simulink model "quadrotor_linear_ADRC"  (R2018b)
settings: Solver=VariableStepAuto  StartTime=0.0  StopTime=300  RelTol=1e-3
InitFcn:
  | %%%%%%%%%%%%%%%%%%%%%%%%%
  | %                     TUNABLE PARAMETERS                 %
  | %    (ORDER, SETTLING TIME, ESO GAIN AND B0)  %
  | %%%%%%%%%%%%%%%%%%%%%%%%%
  | order = 2;                     % ADRC order
  | ts = 5;                        % Desired settling time
  | b0 = 1;                         % b0 parameter
  | eso_gain = 8;                % ESO Dynamic related to closed-loop poles
  | 
  | %%%%%%%%%%%%%%%%%%%%%%%%%
  | %                                 ADRC                               %
  | %      (CONTROLLER GAINS AND ESO MATRIXES)    %
  | %%%%%%%%%%%%%%%%%%%%%%%%%
  | s_cl = 4/ts;                           % Closed-loop system poles
  | s_eso = eso_gain * s_cl;        % ESO poles
  | pole = [1 s_cl];                     % Base polynomial to calculate
  |                                            % System characteristic polynomial
  | pole_eso = [1 s_eso];            % Base polynomial to calculate
  |                                            % ESO characteristic polynomial
  | A = zeros(order + 1);            % Matrix A of ESO
  | B = zeros(order + 1, 1);        % Matrix B of ESO
  | C = [1 zeros(1, order)];         % Matrix C of ESO
  | 
  | %%%%%%%%%%%%%%%%%%%%%%%%%%%%%%%%%%%
  | % Here we'll calculate the characteristic polynomials of system and ESO,   %
  | % starting with the base polynomial, and convoluting it until we achieve    %
  | % the system's order.                                                                           %
  | % Also, we'll put the values of A and B matrixes of ESO, filling the             %
  | % diagonal above the main diagonal of A with one's, and putting the value %
  | % b0 on the penultimate value of B matrix, according to ADRC generalized %
  | % model fot Nth order.                                                                          %
  | %%%%%%%%%%%%%%%%%%%%%%%%%%%%%%%%%%%
  | A_sys = pole;
  | A_eso = pole_eso;
  | 
  | for i = 1:order
  |     if i ~= order
  |         A_sys = conv(A_sys, pole);
  |     else
  |         B(i) = b0;
  |     end
  |     A(i,i+1) = 1;
  |     A_eso = conv(A_eso, pole_eso);
  | end
  | 
  | K = [1 A_sys(2:end)];           % Controller gain matrix
  | L = A_eso(2:end)';               % ESO gain matrix
  | 
  | %%%%%%%%%%%%%%%%%%%%%%%%%%%
  | %                         SYSTEM PARAMETERS               %
  | %%%%%%%%%%%%%%%%%%%%%%%%%%%
  | l = 0.232;             % quadrotor arm length
  | b = 3.13e-5;         % propeller lift
  | d = 7.5e-7;           % propeller resistance
  | m = 0.52;             % total quadrotor mass
  | Ix = 6.228e-3;      % Inertia moment X-axis
  | Iy = 6.228e-3;      % Inertia moment Y-axis
  | Iz = 1.121e-2;       % Inertia moment Z-axis
  | Jr = 6e-5;          % Propeller Inertia moment Z-axis
  | Tad = 0.5;        % drag force on the body movement
  | Rad = 0.02;      % drag force on the body rotation
  | g = 9.81;               % gravity
libraries: dspindex x1
settings Model: Creator=root  LastModifiedBy=root

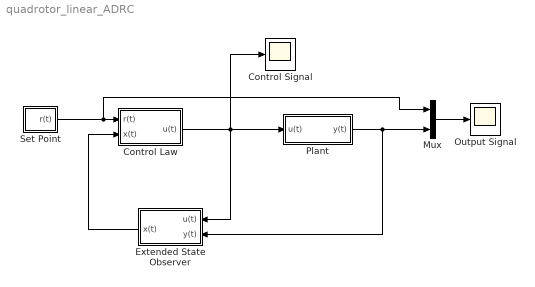
== system quadrotor_linear_ADRC ==
  Control Law : Subsystem
  Control Signal : Scope
  Extended State Observer : Subsystem
  Mux : Mux  Inputs=2
  Output Signal : Scope
  Plant : Subsystem
  Set Point : Subsystem
  wires:
  Set Point/1(r(t)) -> Mux/1, Control Law/1(r(t))
  Mux/1 -> Output Signal/1
  Extended State Observer/1(x(t)) -> Control Law/2(x(t))
  Plant/1(y(t)) -> Extended State Observer/2(y(t)), Mux/2
  Control Law/1(u(t)) -> Control Signal/1, Plant/1(u(t)), Extended State Observer/1("u(t) ")

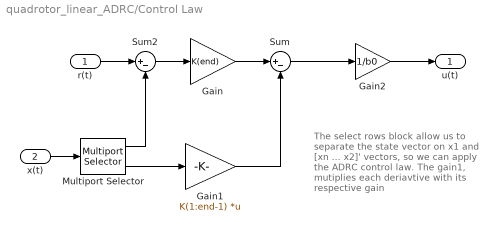
== system quadrotor_linear_ADRC/Control Law ==
  note: The select rows block allow us to separate the state vector on x1 and [xn ... x2]' vectors, so we can apply the ADRC control law. The gain1, mutiplies each deriavtive with its respective gain
  r(t) : Inport
  x(t) : Inport  Port=2
  Gain : Gain  Gain=K(end)  ParamDataTypeStr=Inherit: Inherit from 'Gain'
  Gain1 : Gain  Gain=K(1:end-1)  Multiplication=Matrix(K*u) (u vector)
  Gain2 : Gain  Gain=1/b0
  Multiport Selector : dspindex/Multiport Selector  rowsOrCols=Rows  idxCellArray={ 1, [order+1:-1:2]}  idxErrMode=Clip Index
  Sum : Sum  Inputs=|+-
  Sum2 : Sum  Inputs=|+-
  u(t) : Outport
  wires:
  Gain2/1 -> u(t)/1
  Sum/1 -> Gain2/1
  r(t)/1 -> Sum2/1
  Sum2/1 -> Gain/1
  Gain/1 -> Sum/1
  x(t)/1 -> Multiport Selector/1
  Multiport Selector/1 -> Sum2/2
  Multiport Selector/2 -> Gain1/1
  Gain1/1 -> Sum/2

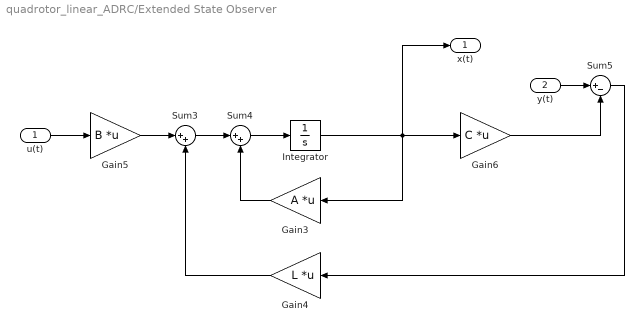
== system quadrotor_linear_ADRC/Extended State Observer ==
  "u(t) " : Inport
  y(t) : Inport  Port=2
  Gain3 : Gain  Gain=A  Multiplication=Matrix(K*u) (u vector)
  Gain4 : Gain  Gain=L  Multiplication=Matrix(K*u) (u vector)
  Gain5 : Gain  Gain=B  Multiplication=Matrix(K*u) (u vector)
  Gain6 : Gain  Gain=C  Multiplication=Matrix(K*u) (u vector)
  Integrator : Integrator
  Sum3 : Sum  Inputs=|++
  Sum4 : Sum  Inputs=|++
  Sum5 : Sum  Inputs=|+-
  x(t) : Outport
  wires:
  Sum4/1 -> Integrator/1
  y(t)/1 -> Sum5/1
  Gain4/1 -> Sum3/2
  Gain5/1 -> Sum3/1
  Gain3/1 -> Sum4/2
  Sum3/1 -> Sum4/1
  Sum5/1 -> Gain4/1
  Gain6/1 -> Sum5/2
  Integrator/1 -> x(t)/1, Gain3/1, Gain6/1
  "u(t) "/1 -> Gain5/1

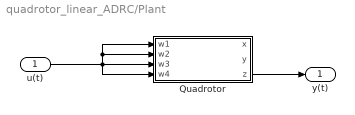
== system quadrotor_linear_ADRC/Plant ==
  u(t) : Inport
  Quadrotor : Subsystem
  y(t) : Outport
  wires:
  u(t)/1 -> Quadrotor/4(w4), Quadrotor/2(w2), Quadrotor/1(w1), Quadrotor/3(w3)
  Quadrotor/3(z) -> y(t)/1

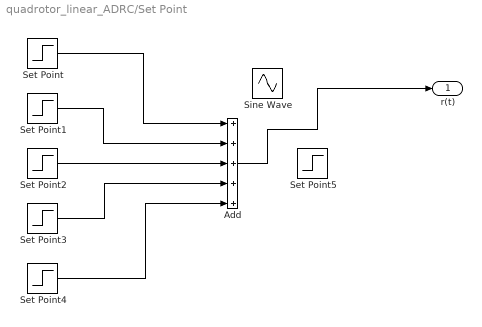
== system quadrotor_linear_ADRC/Set Point ==
  Add : Sum  Inputs=+++++
  Set Point : Step  Time=0  After=10  SampleTime=0
  Set Point1 : Step  Time=50  After=2  SampleTime=0
  Set Point2 : Step  Time=120  After=-1.3  SampleTime=0
  Set Point3 : Step  Time=180  After=3.5  SampleTime=0
  Set Point4 : Step  Time=250  After=-2  SampleTime=0
  Set Point5 : Step  After=20  SampleTime=0
  Sine Wave : Sin  Amplitude=3  Bias=10  SampleTime=0
  r(t) : Outport
  wires:
  Set Point2/1 -> Add/3
  Set Point4/1 -> Add/5
  Set Point3/1 -> Add/4
  Set Point1/1 -> Add/2
  Set Point/1 -> Add/1
  Add/1 -> r(t)/1

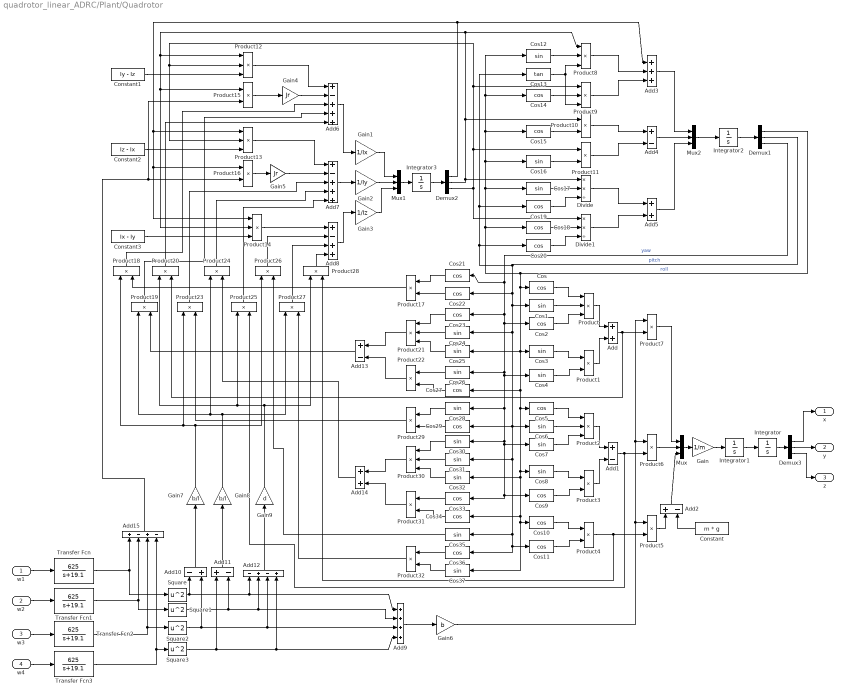
== system quadrotor_linear_ADRC/Plant/Quadrotor ==
  w1 : Inport
  w2 : Inport  Port=2
  w3 : Inport  Port=3
  w4 : Inport  Port=4
  Add : Sum
  Add{1..2,4,11,13} (5 alike) : Sum  Inputs=+-
  Add10 : Sum  Inputs=-+
  Add12 : Sum  Inputs=-+-+
  Add14 : Sum
  Add15 : Sum  Inputs=+-+-
  Add3 : Sum  Inputs=+++
  Add5 : Sum
  Add6 : Sum  Inputs=+-+++
  Add7 : Sum  Inputs=+-+++
  Add8 : Sum  Inputs=+-++
  Add9 : Sum  Inputs=++++
  Constant : Constant  Value=m * g
  Constant1 : Constant  Value=Iy - Iz
  Constant2 : Constant  Value=Iz - Ix
  Constant3 : Constant  Value=Ix - Iy
  Cos{,2,5,9..11,14..15,18..23,27,29,33..34,36} (19 alike) : Trigonometry  Operator=cos
  Cos{1,3..4,6..8,12,16..17,24..26,28,30..32,35,37} (18 alike) : Trigonometry
  Cos13 : Trigonometry  Operator=tan
  Demux1 : Demux  Outputs=3
  Demux2 : Demux  Outputs=3
  Demux3 : Demux  Outputs=3
  Divide : Product  Inputs=**/
  Divide1 : Product  Inputs=**/
  Gain : Gain  Gain=1/m
  Gain1 : Gain  Gain=1/Ix
  Gain2 : Gain  Gain=1/Iy
  Gain3 : Gain  Gain=1/Iz
  Gain4 : Gain  Gain=Jr
  Gain5 : Gain  Gain=Jr
  Gain6 : Gain  Gain=b
  Gain7 : Gain  Gain=b/l
  Gain8 : Gain  Gain=b/l
  Gain9 : Gain  Gain=d
  Integrator{,1..3} (4 alike) : Integrator
  Mux : Mux  Inputs=3
  Mux1 : Mux  Inputs=3
  Mux2 : Mux  Inputs=3
  Product{,2,8..9,12..14,21,30} (9 alike) : Product  Inputs=3
  Product{1,3..7,10..11,15..20,22..29,31..32} (24 alike) : Product
  Square{,1..3} (4 alike) : Math  Operator=square  SaturateOnIntegerOverflow=on
  Transfer Fcn{,1..3} (4 alike) : TransferFcn  Numerator=[625]  Denominator=[1 19.1]
  x : Outport
  y : Outport  Port=2
  z : Outport  Port=3
  wires:
  Product7/1 -> Mux/1
  Cos18/1 -> Divide1/2
  Divide/1 -> Add5/1
  Add2/1 -> Mux/3
  Cos15/1 -> Product10/2
  Product10/1 -> Add4/1
  Cos12/1 -> Product8/2
  Product1/1 -> Add/2
  Product11/1 -> Add4/2
  Product8/1 -> Add3/2
  Demux3/1 -> x/1
  Add3/1 -> Mux2/1
  Product5/1 -> Add2/1
  Cos11/1 -> Product4/2
  Add7/1 -> Gain2/1
  Cos17/1 -> Divide/2
  Product/1 -> Add/1
  Cos8/1 -> Product3/1
  Add12/1 -> Gain9/1
  Cos7/1 -> Product2/3
  Add8/1 -> Gain3/1
  Add5/1 -> Mux2/3
  Gain/1 -> Integrator1/1
  Cos19/1 -> Divide/3
  Product4/1 -> Product5/2, Product28/2
  Integrator/1 -> Demux3/1
  Square1/1 -> Add11/2, Add12/2, Add9/2
  Cos14/1 -> Product9/2
  Demux3/3 -> z/1
  Cos/1 -> Product/1
  Divide1/1 -> Add5/2
  Gain4/1 -> Add6/2
  Cos16/1 -> Product11/2
  Product15/1 -> Gain4/1
  Demux2/2 -> Divide/1, Product8/1, Product14/2, Product15/1, Product12/1, Product10/1
  Product14/1 -> Add8/1
  Gain2/1 -> Mux1/2
  Cos1/1 -> Product/2
  Integrator1/1 -> Integrator/1
  Demux3/2 -> y/1
  Gain6/1 -> Product7/1, Product6/1, Product5/1
  Square2/1 -> Add10/2, Add12/3, Add9/3
  Transfer Fcn2/1 -> Add15/3, Square2/1
  Product6/1 -> Mux/2
  Cos9/1 -> Product3/2
  Add6/1 -> Gain1/1
  Add4/1 -> Mux2/2
  Gain5/1 -> Add7/2
  Integrator2/1 -> Demux1/1
  Add10/1 -> Gain7/1
  Cos4/1 -> Product1/2
  Product3/1 -> Add1/2
  Square/1 -> Add10/1, Add12/1, Add9/1
  Add9/1 -> Gain6/1
  Demux2/3 -> Divide1/1, Product11/1, Product9/1, Product13/2, Product12/2
  Transfer Fcn3/1 -> Square3/1, Add15/4
  Gain3/1 -> Mux1/3
  Product16/1 -> Gain5/1
  Gain1/1 -> Mux1/1
  Constant2/1 -> Product13/3
  Cos10/1 -> Product4/1
  Product2/1 -> Add1/1
  Mux2/1 -> Integrator2/1
  Cos20/1 -> Divide1/3
  Demux1/1 -> Cos18/1, Cos17/1, Cos16/1, Cos14/1, Cos12/1, Cos15/1, Cos25/1, Cos27/1, Cos37/1, Cos10/1, Cos34/1, Cos32/1, Cos8/1, Cos5/1, Cos3/1, Cos/1  "roll"
  Cos2/1 -> Product/3
  Add/1 -> Product20/2, Product7/2
  Constant1/1 -> Product12/3
  Integrator3/1 -> Demux2/1
  Demux2/1 -> Add3/1, Product14/1, Product16/1, Product13/1
  Product12/1 -> Add6/1
  Transfer Fcn1/1 -> Square1/1, Add15/2
  Add11/1 -> Gain8/1
  Constant3/1 -> Product14/3
  Mux/1 -> Gain/1
  Cos3/1 -> Product1/1
  Demux1/3 -> Cos23/1, Cos2/1, Cos26/1, Cos28/1, Cos33/1, Cos9/1, Cos7/1, Cos30/1, Cos4/1, Cos21/1  "yaw"
  Product13/1 -> Add7/1
  Product9/1 -> Add3/3
  Demux1/2 -> Cos20/1, Cos19/1, Cos13/1, Cos1/1, Cos24/1, Cos29/1, Cos35/1, Cos36/1, Cos11/1, Cos31/1, Cos6/1, Cos22/1  "pitch"
  Constant/1 -> Add2/2
  Cos13/1 -> Product9/3, Product8/3
  Mux1/1 -> Integrator3/1
  Cos5/1 -> Product2/1
  Cos6/1 -> Product2/2
  Add1/1 -> Product6/2, Product25/2
  Add15/1 -> Product15/2, Product16/2
  Product18/1 -> Add6/3
  Product19/1 -> Add6/4
  Gain8/1 -> Product24/1, Product19/1, Product27/1
  Gain9/1 -> Product28/1, Product25/1, Product20/1
  Product20/1 -> Add6/5
  Cos21/1 -> Product17/1
  Product17/1 -> Product18/2
  Add13/1 -> Product19/2
  Cos22/1 -> Product17/2
  Product21/1 -> Add13/1
  Product22/1 -> Add13/2
  Cos23/1 -> Product21/1
  Cos24/1 -> Product21/2
  Cos25/1 -> Product21/3
  Cos26/1 -> Product22/1
  Cos27/1 -> Product22/2
  Gain7/1 -> Product18/1, Product23/1, Product26/1
  Product23/1 -> Add7/3
  Product24/1 -> Add7/4
  Product25/1 -> Add7/5
  Product26/1 -> Add8/2
  Product27/1 -> Add8/3
  Product28/1 -> Add8/4
  Cos28/1 -> Product29/1
  Cos29/1 -> Product29/2
  Cos30/1 -> Product30/1
  Product31/1 -> Add14/2
  Cos31/1 -> Product30/2
  Cos33/1 -> Product31/1
  Cos34/1 -> Product31/2
  Product30/1 -> Add14/1
  Cos32/1 -> Product30/3
  Add14/1 -> Product24/2
  Cos35/1 -> Product26/2
  Cos36/1 -> Product32/1
  Cos37/1 -> Product32/2
  Product32/1 -> Product27/2
  Product29/1 -> Product23/2
  Transfer Fcn/1 -> Square/1, Add15/1
  Square3/1 -> Add11/1, Add12/4, Add9/4
  w1/1 -> Transfer Fcn/1
  w2/1 -> Transfer Fcn1/1
  w3/1 -> Transfer Fcn2/1
  w4/1 -> Transfer Fcn3/1
